simulink model "Mod4_1"  (Simulink 7.4)
settings: Solver=FixedStepDiscrete  SolverMode=SingleTasking  StartTime=0.0  StopTime=inf  MaxStep=1e-6  RelTol=1e-3  AbsTol=1e-6
InitFcn:
  | Fs=1.024e6;
  | OSR=128;
  | a1=1/3;
  | a2=3/25;
  | a3=1/10;
  | a4=1/25;
  | b1=1;
  | b2=0.8;
  | alpha=1/5;
  | beta=1/2;
undefined symbols (not defined in the file or in its folder): One, sided
libraries: dspbuff3 x3, dspmlti4 x3, simulink x2, dspobslib x2, dspspect3 x2, dspsnks4 x2, commsynccomp2 x1, dsparch4 x1, dspadpt3 x1, dspsigops x1, dspstat3 x1
settings Model: Creator=don  LastModifiedBy=Dick  ExtModeTrigMode=oneshot  ExtModeArmWhenConnect=off
settings DataIOCC: LimitDataPoints=off  SaveOutput=off  SaveTime=off  SignalLoggingName=sigsOut
settings OptimizationCC: BlockReduction=off  BooleanDataType=off  InitFltsAndDblsToZero=on
settings DebuggingCC: SaveWithParameterizedLinksMsg=none  SignalResolutionControl=TryResolveAllWithWarning  SolverPrmCheckMsg=none  MultiTaskDSMMsg=warning  MultiTaskCondExecSysMsg=none  IntegerOverflowMsg=none  StrictBusMsg=None
settings HardwareCC: TargetUnknown=on
settings RTWCC: IncludeERTFirstTime=on
settings GRTTargetCC: TargetFcnLib=ansi_tfl_tmw.mat

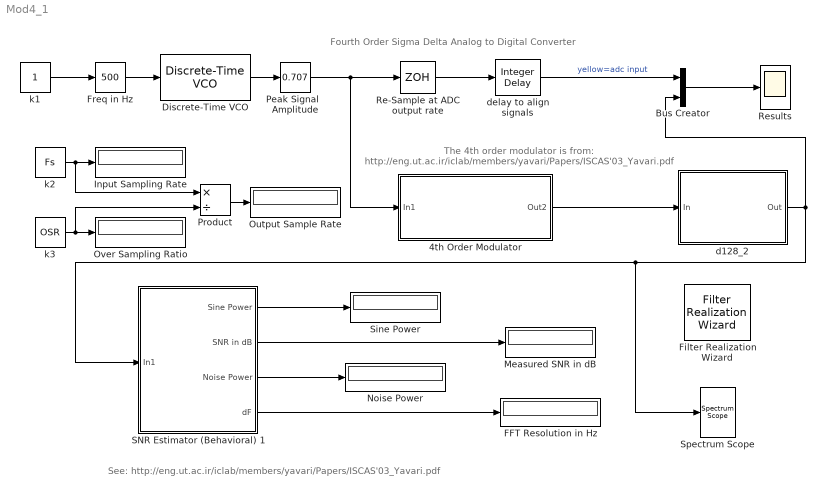
== system Mod4_1 ==
  note: The 4th order modulator is from:
      | http://eng.ut.ac.ir/iclab/members/yavari/Papers/ISCAS'03_Yavari.pdf
  note: Fourth Order Sigma Delta Analog to Digital Converter
  note: See: http://eng.ut.ac.ir/iclab/members/yavari/Papers/ISCAS'03_Yavari.pdf
  4th Order Modulator : Subsystem
  Bus Creator : BusCreator  Inputs=2
  Discrete-Time VCO : commsynccomp2/Discrete-Time VCO  SystemSampleTime=-1  Ac=1  Fc=0  Kc=1  Ph=pi/2  ts=1/Fs
  FFT Resolution in Hz : Display
  Filter Realization Wizard : dsparch4/Filter Realization Wizard  SystemSampleTime=-1
  Freq in Hz : simulink/Math Operations/Slider Gain  SystemSampleTime=-1  low=0  gain=500  high=4000
  Input Sampling Rate : Display
      settings: Decimation=1000
  Measured SNR in dB : Display
  Noise Power : Display
  Output Sample Rate : Display
      settings: Decimation=1000
  Over Sampling Ratio : Display
      settings: Decimation=1000
  Peak Signal   Amplitude : simulink/Math Operations/Slider Gain  SystemSampleTime=-1  low=0  gain=0.707  high=1
  Product : Product  Inputs=*/  OutDataType=fixdt(1, 16)  OutScaling=2^0  RndMeth=Zero
  Re-Sample at ADC output rate : ZeroOrderHold  SampleTime=OSR/Fs
  Results : Scope
      settings: TimeRange=0.02  YMin=-0.8  YMax=0.8  DataFormat=Array
  SNR Estimator (Behavioral) 1 : Subsystem  mask{Frame=256, Pcnt_Nyquist=100, Navg=1, Ymax=-50, Ymin=-140, Hold_Off=260, ON_FFT_LINE=off}
      mask prompts: Frame "Input Frame Size"; Pcnt_Nyquist "Percentage of Fs/2 to use in noise power measurement"; Navg "Number of Averages"; Ymax "Noise Plot Ymax in dB"; Ymin "Noise Plot Ymin in dB"; Hold_Off "Calculation Hold Off in SAMPLES"; ON_FFT_LINE "Check this box if the signal is on an FFT Analysis Line."
      mask Display:
      | disp('SNR \n Measurement')
      | port_label('Input',1,'In')
      | port_label('Output',1,'Sine Power')
      | port_label('Output',2,'SNR in dB')
      | port_label('Output',3,'Noise Power')
      | port_label('Output',4,'FFT Line Freq')
  "Sine Power " : Display
  Spectrum Scope : dspsnks4/Spectrum Scope  DialogController=dspdialog.SpectrumScope  DialogControllerArgs=DataTag2  SystemSampleTime=-1  ScopeProperties=off  Domain=Frequency  HorizSpan=1  UseBuffer=on  BufferSize=1024  Overlap=0  inpFftLenInherit=off  FFTlength=128  numAvg=1  DisplayProperties=off  AxisGrid=on  Memory=off  FrameNumber=on  AxisLegend=off  AxisZoom=off  OpenScopeAtSimStart=on  OpenScopeImmediately=off  FigPos=[281 33 319 232]  AxisProperties=on  XUnits=Hertz  XRange=One-sided ([0...Fs/2])  XDisplay=0  InheritXIncr=on  XIncr=1.0  XLabel=Samples  XLimit=Auto  YUnits=dBW  XMax=1  XMin=0  YLabel=Magnitude, dB  LineProperties=off  wintypeSpecScope=Hann  RsSpecScope=50  betaSpecScope=5  winsampSpecScope=Periodic  XAxisParamsVer=6.9
      settings: YMin=-140  YMax=0
  d128_2 : Subsystem  Tag=BlockMethodSubSystem
  delay to align signals : dspobslib/Integer Delay  delay=9  ic=0  reset_popup=None
  k1 : Constant  OutDataType=fixdt(1, 16)  OutScaling=2^0
  k2 : Constant  Value=Fs  OutDataType=fixdt(1, 16)  OutScaling=2^0
  k3 : Constant  Value=OSR  OutDataType=fixdt(1, 16)  OutScaling=2^0
  wires:
  Discrete-Time VCO/1 -> Peak Signal   Amplitude/1
  Peak Signal   Amplitude/1 -> Re-Sample at ADC output rate/1, 4th Order Modulator/1(In1)
  Freq in Hz/1 -> Discrete-Time VCO/1
  k1/1 -> Freq in Hz/1
  Bus Creator/1 -> Results/1
  Re-Sample at ADC output rate/1 -> delay to align signals/1
  delay to align signals/1 -> Bus Creator/1  "yellow=adc input"
  k2/1 -> Input Sampling Rate/1, Product/1
  k3/1 -> Over Sampling Ratio/1, Product/2
  Product/1 -> Output Sample Rate/1
  d128_2/1(Out) -> Bus Creator/2, Spectrum Scope/1, SNR Estimator (Behavioral) 1/1(In1)
  SNR Estimator (Behavioral) 1/2(SNR in dB) -> Measured SNR in dB/1
  SNR Estimator (Behavioral) 1/1(Sine Power) -> "Sine Power "/1
  SNR Estimator (Behavioral) 1/3(Noise Power) -> Noise Power/1
  SNR Estimator (Behavioral) 1/4(dF) -> FFT Resolution in Hz/1
  4th Order Modulator/1(Out2) -> d128_2/1(In)

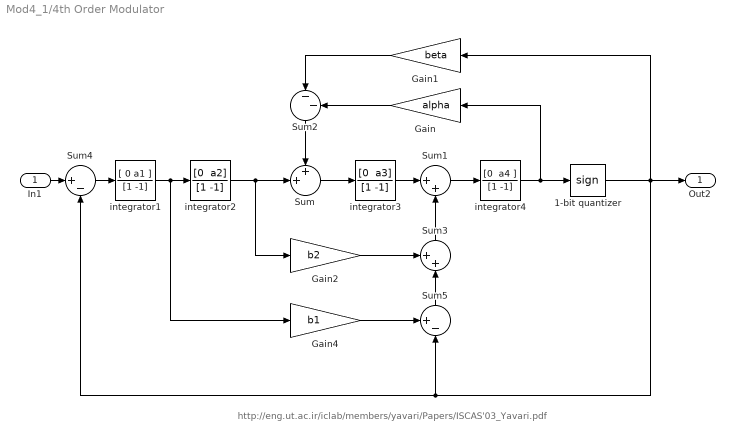
== system Mod4_1/4th Order Modulator ==
  note: http://eng.ut.ac.ir/iclab/members/yavari/Papers/ISCAS'03_Yavari.pdf
  In1 : Inport
  1-bit quantizer : Signum
  Gain : Gain  Gain=alpha  ParameterDataType=fixdt(1, 16)  ParameterScaling=2^0  OutDataType=fixdt(1, 16)  OutScaling=2^0
  Gain1 : Gain  Gain=beta  ParameterDataType=fixdt(1, 16)  ParameterScaling=2^0  OutDataType=fixdt(1, 16)  OutScaling=2^0
  Gain2 : Gain  Gain=b2  ParameterDataType=fixdt(1, 16)  ParameterScaling=2^0  OutDataType=fixdt(1, 16)  OutScaling=2^0
  Gain4 : Gain  Gain=b1  ParameterDataType=fixdt(1, 16)  ParameterScaling=2^0  OutDataType=fixdt(1, 16)  OutScaling=2^0
  Sum : Sum  Inputs=++|  OutDataType=sfix(16)  OutScaling=2^0  SaturateOnIntegerOverflow=on  InputSameDT=on  OutDataTypeStr=Inherit: Same as first input
  Sum1 : Sum  Inputs=|++  OutDataType=sfix(16)  OutScaling=2^0  SaturateOnIntegerOverflow=on  InputSameDT=on  OutDataTypeStr=Inherit: Same as first input
  Sum2 : Sum  Inputs=|--  OutDataType=sfix(16)  OutScaling=2^0  SaturateOnIntegerOverflow=on  InputSameDT=on  OutDataTypeStr=Inherit: Same as first input
  Sum3 : Sum  Inputs=++|  OutDataType=sfix(16)  OutScaling=2^0  SaturateOnIntegerOverflow=on  InputSameDT=on  OutDataTypeStr=Inherit: Same as first input
  Sum4 : Sum  Inputs=|+-  OutDataType=sfix(16)  OutScaling=2^0  SaturateOnIntegerOverflow=on  InputSameDT=on  OutDataTypeStr=Inherit: Same as first input
  Sum5 : Sum  Inputs=+-|  OutDataType=sfix(16)  OutScaling=2^0  SaturateOnIntegerOverflow=on  InputSameDT=on  OutDataTypeStr=Inherit: Same as first input
  integrator1 : DiscreteFilter  Numerator=[ 0 a1 ]  Denominator=[1 -1]
  integrator2 : DiscreteFilter  Numerator="[0  a2]"  Denominator=[1 -1]
  integrator3 : DiscreteFilter  Numerator="[0  a3]"  Denominator=[1 -1]
  integrator4 : DiscreteFilter  Numerator="[0  a4 ]"  Denominator=[1 -1]
  Out2 : Outport
  wires:
  1-bit quantizer/1 -> Gain1/1, Sum4/2, Sum5/2, Out2/1
  integrator3/1 -> Sum1/1
  Sum1/1 -> integrator4/1
  integrator4/1 -> 1-bit quantizer/1, Gain/1
  Sum2/1 -> Sum/1
  Gain/1 -> Sum2/2
  Gain1/1 -> Sum2/1
  Sum/1 -> integrator3/1
  integrator2/1 -> Sum/2, Gain2/1
  integrator1/1 -> integrator2/1, Gain4/1
  Sum3/1 -> Sum1/2
  Gain2/1 -> Sum3/1
  Sum4/1 -> integrator1/1
  In1/1 -> Sum4/1
  Sum5/1 -> Sum3/2
  Gain4/1 -> Sum5/1

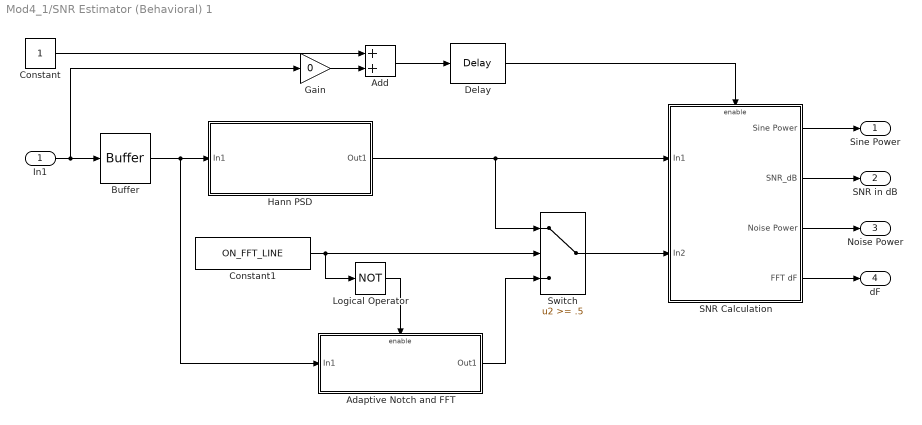
== system Mod4_1/SNR Estimator (Behavioral) 1 ==
  In1 : Inport
  Adaptive Notch and FFT : Subsystem  TreatAsAtomicUnit=on
  Add : Sum  OutDataType=fixdt(1, 16)  OutScaling=2^-10
  Buffer : dspbuff3/Buffer  N=Frame  V=0  ic=0
  Constant : Constant  OutDataType=fixdt(1, 16)  OutScaling=2^0
  Constant1 : Constant  Value=ON_FFT_LINE  OutDataTypeMode=boolean  OutDataType=fixdt(1, 16)  OutScaling=2^0  OutDataTypeStr=boolean
  Delay : dspsigops/Delay  dly_unit=Samples  delay=Hold_Off  ic_detail=off  dif_ic_for_ch=off  dif_ic_for_dly=off  ic=0  reset_popup=None
  Gain : Gain  Gain=0  ParameterDataType=fixdt(1, 16)  ParameterScaling=2^0  OutDataType=fixdt(1, 16)  OutScaling=2^0
  Hann PSD : Subsystem
  Logical Operator : Logic  Operator=NOT  AllPortsSameDT=off  OutDataTypeMode=boolean  LogicDataType=fixdt(0, 8)  OutDataTypeStr=boolean
  SNR Calculation : Subsystem
  Switch : Switch  Threshold=.5  OutDataType=fixdt(1, 16)  OutScaling=2^0
  Sine Power : Outport
  SNR in dB : Outport  Port=2
  Noise Power : Outport  Port=3
  dF : Outport  Port=4
  wires:
  In1/1 -> Buffer/1, Gain/1
  SNR Calculation/2(SNR_dB) -> SNR in dB/1
  Hann PSD/1(Out1) -> SNR Calculation/1(In1), Switch/1
  Buffer/1 -> Hann PSD/1(In1), Adaptive Notch and FFT/1(In1)
  SNR Calculation/1(Sine Power) -> Sine Power/1
  Switch/1 -> SNR Calculation/2(In2)
  SNR Calculation/3(Noise Power) -> Noise Power/1
  Delay/1 -> SNR Calculation/Enable
  Adaptive Notch and FFT/1(Out1) -> Switch/3
  Constant1/1 -> Switch/2, Logical Operator/1
  Logical Operator/1 -> Adaptive Notch and FFT/Enable
  SNR Calculation/4(FFT dF) -> dF/1
  Add/1 -> Delay/1
  Constant/1 -> Add/1
  Gain/1 -> Add/2

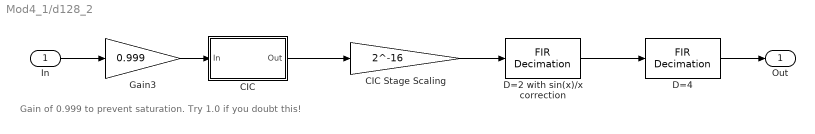
== system Mod4_1/d128_2 ==
  note: Gain of 0.999
      |  to prevent saturation.
      | Try 1.0 if you doubt this!
  In : Inport
  CIC : Subsystem  Tag=BlockMethodSubSystem
  CIC Stage Scaling : Gain  Gain=2^-16  ParameterDataType=fixdt(1, 16)  ParameterScaling=2^0  OutDataTypeMode=double  OutDataType=fixdt(1, 16)  OutScaling=2^0  OutDataTypeStr=double
  D=2 with sin(x)/x correction : dspmlti4/FIR Decimation  Tag=BlockMethodSubSystem  DialogController=dspdialog.FIRDecimation  DialogControllerArgs=DataTag3  h=[0.000549322570782159 0.0028188201427819 0.00605408312993028 0.00388745313496409 -0.0121134249050654 -0.0371670852364025 -0.0412525748188521 0.0145135665847005 0.134839839295902 0.264505645586551 0.320972309879795 0.264505645586551 0.134839839295902 0.0145135665847005 -0.0412525748188521 -0.0371670852364025 -0.0121134249050654 0.00388745313496409 0.00605408312993028 0.0028188201427819 0.000549322570782159]  D=2  filtStruct=Direct form  framing=Maintain input frame size  outputBufInitCond=0  roundingMode=Floor  overflowMode=off  FilterSource=Specify via dialog  FilterObject=Hm_firdecim
  D=4 : dspmlti4/FIR Decimation  Tag=BlockMethodSubSystem  DialogController=dspdialog.FIRDecimation  DialogControllerArgs=DataTag4  h=[3.91622882568566e-005 6.87965858042108e-005 -4.54214374064863e-005 -0.000494371495641253 -0.00130180300923401 -0.00208967903904167 -0.00212227242054207 -0.000820466891279789 0.00150204580522739 0.00336930831020411 0.00293785704853453 -0.000377156856911545 -0.00470730589029979 -0.00641725180832836 -0.00285434238807273 0.00468881704747952 0.0106481610663031 0.00886595641260817 -0.00177682957707149 -0.0144760924096176 -0.0180887636371107 -0.00603326390232397 0.0159987454589339 0.0309930177585429 0.0221515825094605 -0.011846123967549 -0.04979943488328 -0.0572170491759349 -0.00847489358036981 0.0923226139783473 0.207458472082029 0.283964644704709 0.283964644704709 0.207458472082029 0.0923226139783473 -0.00847489358036981 -0.0572170491759349 -0.04979943488328 -0.011846123967549 0.0221515825094605 0.0309930177585429 0.0159987454589339 -0.00603326390232397 -0.0180887636371107 -0.0144760924096176 -0.00177682957707149 0.00886595641260817 0.0106481610663031 0.00468881704747952 -0.00285434238807273 -0.00641725180832836 -0.00470730589029979 -0.000377156856911545 0.00293785704853453 0.00336930831020411 0.00150204580522739 -0.000820466891279789 -0.00212227242054207 -0.00208967903904167 -0.00130180300923401 -0.000494371495641253 -4.54214374064863e-005 6.87965858042108e-005 3.91622882568566e-005]  D=4  filtStruct=Direct form  framing=Maintain input frame size  outputBufInitCond=0  roundingMode=Floor  overflowMode=off  FilterSource=Specify via dialog  FilterObject=Hm_firdecim
  Gain3 : Gain  Gain=0.999  ParameterDataType=fixdt(1, 16)  ParameterScaling=2^0  OutDataType=fixdt(1, 16)  OutScaling=2^0
  Out : Outport
  wires:
  In/1 -> Gain3/1
  CIC/1(Out) -> CIC Stage Scaling/1
  D=2 with sin(x)/x correction/1 -> D=4/1
  D=4/1 -> Out/1
  CIC Stage Scaling/1 -> D=2 with sin(x)/x correction/1
  Gain3/1 -> CIC/1(In)

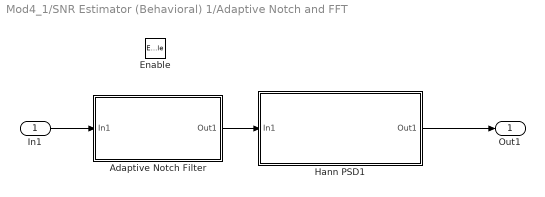
== system Mod4_1/SNR Estimator (Behavioral) 1/Adaptive Notch and FFT ==
  In1 : Inport  OutDataType=fixdt(1, 16)  OutScaling=2^0
  Enable : EnablePort
  Adaptive Notch Filter : Subsystem
  Hann PSD1 : Subsystem
  Out1 : Outport  OutDataType=fixdt(1, 16)  OutScaling=2^0
  wires:
  Adaptive Notch Filter/1(Out1) -> Hann PSD1/1(In1)
  Hann PSD1/1(Out1) -> Out1/1
  In1/1 -> Adaptive Notch Filter/1(In1)

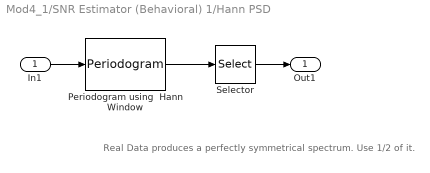
== system Mod4_1/SNR Estimator (Behavioral) 1/Hann PSD ==
  note: Real Data produces a perfectly
      | symmetrical spectrum.
      | Use 1/2 of it.
  In1 : Inport
  Periodogram using  Hann Window : dspspect3/Periodogram  SystemSampleTime=-1  measurement=Mean-square spectrum  wintype=Hann  Rs=RsSpecScope  beta=betaSpecScope  winsamp=Periodic  inheritFFT=on  fftsize=FFTlength  navg=Navg  inheritTs=on  Ts=1
  Selector : Selector  InputPortWidth=Frame  IndexOptions=Index vector (dialog)  Indices=[1: Frame/2]  OutputSizes=1
  Out1 : Outport
  wires:
  Selector/1 -> Out1/1
  Periodogram using  Hann Window/1 -> Selector/1
  In1/1 -> Periodogram using  Hann Window/1

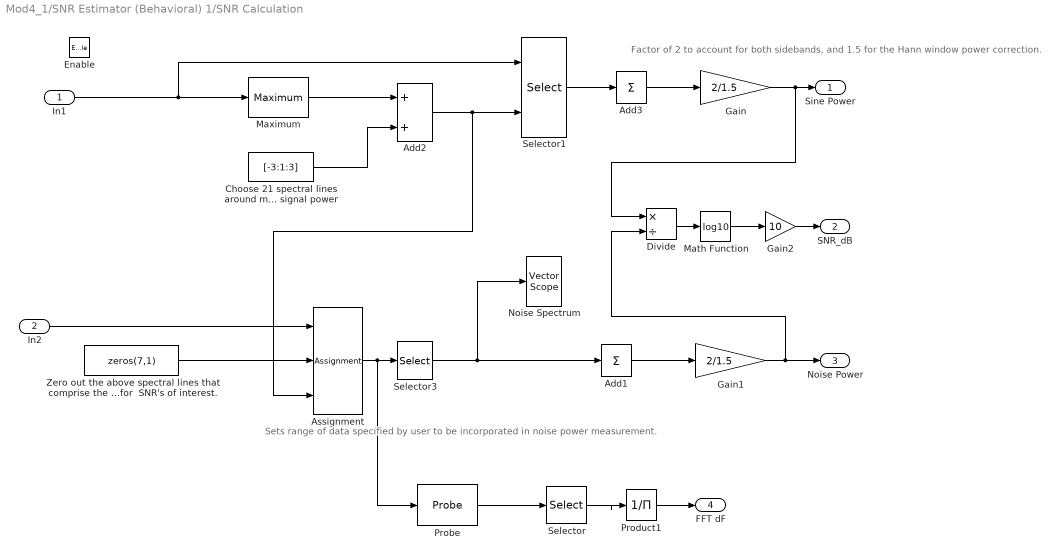
== system Mod4_1/SNR Estimator (Behavioral) 1/SNR Calculation ==
  note: Factor of 2 to account for both sidebands,
      | and 1.5 for the Hann window
      | power correction.
  note: Sets range of data
      | specified by user to be
      |  incorporated in
      | noise power measurement.
  In1 : Inport
  In2 : Inport  Port=2
  Enable : EnablePort
  Add1 : Sum  Inputs=+  OutDataType=fixdt(1, 16)  OutScaling=2^-10
  Add2 : Sum  OutDataType=fixdt(1, 16)  OutScaling=2^-10
  Add3 : Sum  Inputs=+  OutDataType=fixdt(1, 16)  OutScaling=2^-10
  Assignment : Assignment  IndexOptions=Index vector (port)  Indices=1  OutputSizes=1
  Choose 21 spectral lines around max to  estimate signal power : Constant  Value=[-3:1:3]  OutDataType=fixdt(1, 16)  OutScaling=2^0
  Divide : Product  Inputs=*/  OutDataType=fixdt(1, 16)  OutScaling=2^-10
  Gain : Gain  Gain=2/1.5  ParameterDataType=fixdt(1, 16)  ParameterScaling=2^0  OutDataType=fixdt(1, 16)  OutScaling=2^0
  Gain1 : Gain  Gain=2/1.5  ParameterDataType=fixdt(1, 16)  ParameterScaling=2^0  OutDataType=fixdt(1, 16)  OutScaling=2^0
  Gain2 : Gain  Gain=10  ParameterDataType=fixdt(1, 16)  ParameterScaling=2^0  OutDataType=fixdt(1, 16)  OutScaling=2^0
  Math Function : Math  Operator=log10  OutDataType=fixdt(1, 16)  OutScaling=2^0  SaturateOnIntegerOverflow=on
  Maximum : dspstat3/Maximum  DialogController=dspDDGCreate  DialogControllerArgs=DataTag0  fcn=Index  reset=None  indexBase=One  operateOver=Each column  Dimension=1  colComp=on  operation=maximum  roiEnable=off  roiType=Rectangles  roiPortion=Entire ROI  roiOutput=Individual statistics for each ROI  roiFlag=off  accumDataTypeStr=Inherit: Same as product output  accumLastDataTypeStr=Inherit: Same as product output  roundingMode=Floor  overflowMode=off
  Noise Spectrum : dspsnks4/Vector Scope  DialogController=dspdialog.VectorScope  DialogControllerArgs=DataTag1  ScopeProperties=on  Domain=Frequency  HorizSpan=1  DisplayProperties=off  AxisGrid=on  Memory=off  FrameNumber=on  AxisLegend=off  AxisZoom=off  OpenScopeAtSimStart=on  OpenScopeImmediately=off  FigPos=[755 36 259 173]  AxisProperties=off  XUnits=Hertz  XRange=[0...Fs]  InheritXIncr=on  XIncr=1  XLabel=Time  XLimit=Auto  XMin=0  XMax=50000  XStart=0  YUnits=dB  YLabel=dBW  LineProperties=off  XAxisParamsVer=6.9
      settings: YMin=Ymin  YMax=Ymax
  Probe : Probe  ProbeWidth=off  ProbeComplexSignal=off
  Product1 : Product  Inputs=/  OutDataType=fixdt(1, 16)  OutScaling=2^0  RndMeth=Zero
  Selector : Selector  InputPortWidth=2  IndexOptions=Index vector (dialog)  Indices=1  OutputSizes=1
  Selector1 : Selector  InputPortWidth=Frame/2  IndexOptions=Index vector (port)  Indices=[1: Frame/2]  OutputSizes=1
  Selector3 : Selector  InputPortWidth=Frame/2  IndexOptions=Index vector (dialog)  Indices=[1: round(Pcnt_Nyquist*Frame/200)]  OutputSizes=1
  "Zero out the above spectral lines that comprise the signal. Zeroing should not induce any significant error for  SNR's of interest. " : Constant  Value=zeros(7,1)  OutDataType=fixdt(1, 16)  OutScaling=2^0
  Sine Power : Outport
  SNR_dB : Outport  Port=2
  Noise Power : Outport  Port=3
  FFT dF : Outport  Port=4
  wires:
  "Zero out the above spectral lines that comprise the signal. Zeroing should not induce any significant error for  SNR's of interest. "/1 -> Assignment/2
  Add1/1 -> Gain1/1
  Add3/1 -> Gain/1
  Divide/1 -> Math Function/1
  Math Function/1 -> Gain2/1
  Maximum/1 -> Add2/1
  Choose 21 spectral lines around max to  estimate signal power/1 -> Add2/2
  Add2/1 -> Selector1/2, Assignment/3
  Selector1/1 -> Add3/1
  Selector3/1 -> Add1/1, Noise Spectrum/1
  In2/1 -> Assignment/1
  In1/1 -> Maximum/1, Selector1/1
  Gain2/1 -> SNR_dB/1
  Gain/1 -> Divide/1, Sine Power/1
  Gain1/1 -> Divide/2, Noise Power/1
  Assignment/1 -> Selector3/1, Probe/1
  Probe/1 -> Selector/1
  Selector/1 -> Product1/1
  Product1/1 -> FFT dF/1

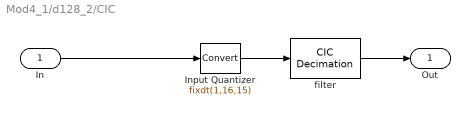
== system Mod4_1/d128_2/CIC ==
  In : Inport
  Input Quantizer : DataTypeConversion  OutDataTypeMode=Specify via dialog  OutDataType=fixdt(1,16,15)  OutDataTypeStr=fixdt(1,16,15)  RndMeth=Round  SaturateOnIntegerOverflow=on
  filter : dspmlti4/CIC Decimation  DialogController=dspdialog.CICDecimation  filtFrom=Dialog  filtobj=Hm_decim  ftype=Decimator  R=16  M=1  N=4  filterInternals=Full precision  BPS=[32 32 32 32 32 32 32 32]  FLPS=[15 15 15 15 15 15 15 15]  outputWordLength=32  outputFracLength=15  launchFVT=off  framing=Maintain input frame rate
  Out : Outport
  wires:
  In/1 -> Input Quantizer/1
  Input Quantizer/1 -> filter/1
  filter/1 -> Out/1

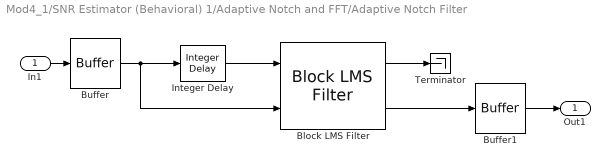
== system Mod4_1/SNR Estimator (Behavioral) 1/Adaptive Notch and FFT/Adaptive Notch Filter ==
  In1 : Inport
  Block LMS Filter : dspadpt3/Block LMS Filter  algo=Block LMS  L=20  N=64  stepflag=Dialog  mu=0.005  leakage=.99999  addnparflag=on  ic=0  Adapt=off  resetflag=None  weights=off
  Buffer : dspbuff3/Buffer  N=64  V=0  ic=0
  Buffer1 : dspbuff3/Buffer  N=Frame  V=0  ic=0
  Integer Delay : dspobslib/Integer Delay  delay=10  ic=0  reset_popup=None
  Terminator : Terminator
  Out1 : Outport
  wires:
  Block LMS Filter/1 -> Terminator/1
  Block LMS Filter/2 -> Buffer1/1
  Buffer1/1 -> Out1/1
  In1/1 -> Buffer/1
  Buffer/1 -> Block LMS Filter/2, Integer Delay/1
  Integer Delay/1 -> Block LMS Filter/1

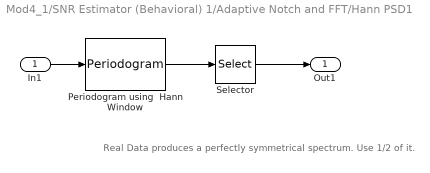
== system Mod4_1/SNR Estimator (Behavioral) 1/Adaptive Notch and FFT/Hann PSD1 ==
  note: Real Data produces a perfectly
      | symmetrical spectrum.
      | Use 1/2 of it.
  In1 : Inport
  Periodogram using  Hann Window : dspspect3/Periodogram  SystemSampleTime=-1  measurement=Mean-square spectrum  wintype=Hann  Rs=RsSpecScope  beta=betaSpecScope  winsamp=Periodic  inheritFFT=on  fftsize=FFTlength  navg=Navg  inheritTs=on  Ts=1
  Selector : Selector  InputPortWidth=Frame  IndexOptions=Index vector (dialog)  Indices=[1: Frame/2]  OutputSizes=1
  Out1 : Outport
  wires:
  In1/1 -> Periodogram using  Hann Window/1
  Periodogram using  Hann Window/1 -> Selector/1
  Selector/1 -> Out1/1
